simulink model "prelab3"  (R2017a)
settings: Solver=ode3  StartTime=0.0  StopTime=5  FixedStep=0.01  RelTol=1e-3
values from neighbouring files (symbols this model uses):
  A = [0 1; 0 (K_t* K_m * K_g^2) / den]    [lab3.m]
  B = [0; (r * K_t * K_g) / den]    [lab3.m]
  C = [1 0]    [lab3.m]
  D = 0    [lab3.m]
  K = 15    [lab3.m]
settings Model: Creator=trey  LastModifiedBy=trey

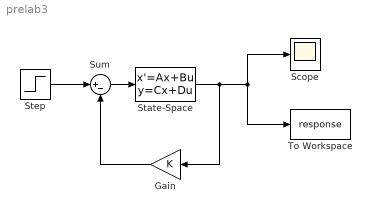
== system prelab3 ==
  Gain : Gain  Gain=K
  Scope : Scope
  State-Space : StateSpace  A=A  B=B  C=C  D=D  X0=0
  Step : Step  Time=0  SampleTime=0
  Sum : Sum  Inputs=|+-
  To Workspace : ToWorkspace  VariableName=response  SaveFormat=Timeseries  SampleTime=-1
  wires:
  Step/1 -> Sum/1
  Sum/1 -> State-Space/1
  State-Space/1 -> Gain/1, To Workspace/1, Scope/1
  Gain/1 -> Sum/2
